simulink model "Part_2_SH_N"  (R2018b)
settings: Solver=VariableStepAuto  StartTime=0.0  StopTime=20.0  MaxStep=0.2  RelTol=1e-3  EnableMultiTasking=on
InitFcn:
  | valve_orifice_area = 0.16;
  | x0 = 0.8;
undefined symbols (not defined in the file): sigbuilder_block
libraries: fl_lib x28, nesl_utility x9, simulink x1
CloseFcn:
  | try,close(h1_sh_power_steering),end
  | clear h1_sh_power_steering
  | try,close(h2_sh_power_steering),end
  | clear h2_sh_power_steering
  | 
  | 
  | clear simlog_sh_power_steering
Description:
  | Power-Assisted Steering Mechanism
  | 
  | Copyright 2008-2018 The MathWorks, Inc.
settings Model: ExtModeAutoUpdateStatusClock=off  Creator=MathWorks  LastModifiedBy=rabia.sehab
settings DataIOCC: LimitDataPoints=on  MaxDataPoints=10000  SaveFormat=Array  SignalLoggingSaveFormat=ModelDataLogs  SignalLoggingName=logsout_sh_power_steering
settings OptimizationCC: ExpressionDepthLimit=2147483647  InitFltsAndDblsToZero=on  LifeSpan=inf
settings DebuggingCC: SaveWithParameterizedLinksMsg=none  UnderspecifiedInitializationDetection=Classic  MergeDetectMultiDrivingBlocksExec=none  SignalResolutionControl=TryResolveAllWithWarning  FcnCallInpInsideContextMsg=warning  AllowSymbolicDim=off  StateNameClashWarn=warning  SFUnexpectedBacktrackingDiag=warning  SFNoUnconditionalDefaultTransitionDiag=warning  SFExecutionAtInitializationDiag=none
settings HardwareCC: ProdBitPerPointer=32  ProdBitPerSizeT=32  ProdBitPerPtrDiffT=32  ProdLargestAtomicFloat=None  ProdIntDivRoundTo=Undefined  ProdEndianess=Unspecified  ProdWordSize=32  ProdHWDeviceType=32-bit Generic
settings ModelReferenceCC: PropagateSignalLabelsOutOfModel=off
settings SFSimCC: SimUseLocalCustomCode=off
settings RTWCC: RTWUseLocalCustomCode=off
settings CodeAppCC: StateflowObjectComments=on
settings GRTTargetCC: TargetFcnLib=ansi_tfl_tmw.mat  TargetLangStandard=C89/C90 (ANSI)  GeneratePreprocessorConditionals=Disable all  CombineOutputUpdateFcns=off  GRTInterface=on
settings ConfigComp: CovMetricSettings=dw  CovHtmlReporting=on  CovSaveCumulativeToWorkspaceVar=on  CovSaveSingleToWorkspaceVar=on  CovExternalEMLEnable=off
settings SimscapeCC: SimscapeLogType=all  SimscapeLogSimulationStatistics=on  SimscapeLogOpenViewer=on  SimscapeLogName=simlog_sh_power_steering  SimscapeLogLimitData=off  SimscapeLogDataHistory=10000

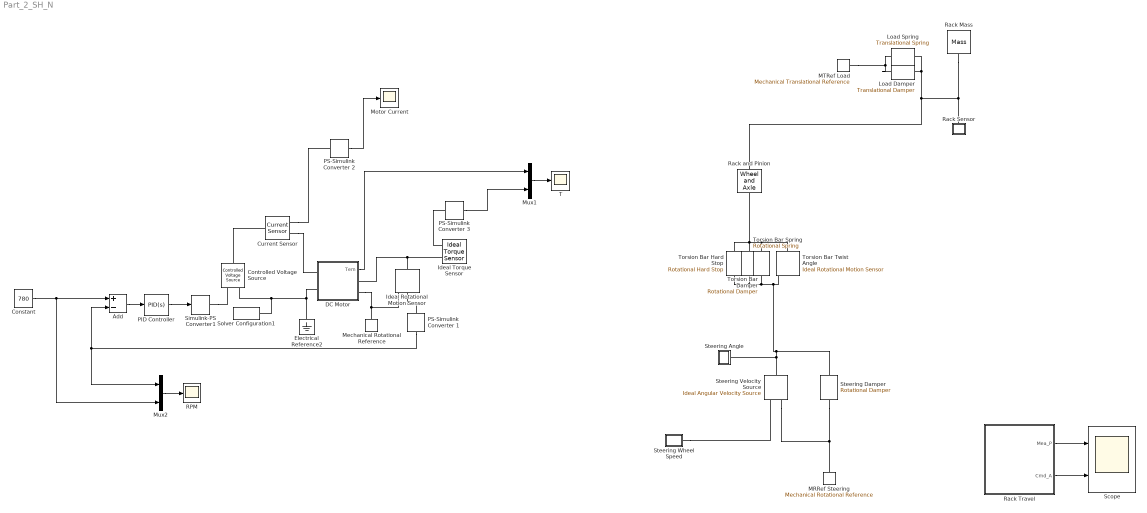
== system Part_2_SH_N ==
  Add : Sum  Inputs=+-
  Constant : Constant  Value=780
  Controlled Voltage Source : fl_lib/Electrical/Electrical Sources/Controlled Voltage Source
  Current Sensor : fl_lib/Electrical/Electrical Sensors/Current Sensor
  DC Motor : Subsystem
  Electrical Reference2 : fl_lib/Electrical/Electrical Elements/Electrical Reference
  Ideal Rotational Motion Sensor : fl_lib/Mechanical/Mechanical Sensors/Ideal Rotational Motion Sensor  offset=0 rad
  Ideal Torque Sensor : fl_lib/Mechanical/Mechanical Sensors/Ideal Torque Sensor
  Load Damper : fl_lib/Mechanical/Translational Elements/Translational Damper  Tag=Factory Generic  D=284 N/(m/s)  v_specify=off  v_priority=High  v=0 m/s  v_nominal_specify=off  v_nominal_unit=m/s  v_nominal_value=1  f_specify=off  f_priority=High  f=0 N  f_nominal_specify=off  f_nominal_unit=N  f_nominal_value=1
  Load Spring : fl_lib/Mechanical/Translational Elements/Translational Spring  Tag=Factory Generic  spr_rate=4450 N/m  v_specify=off  v_priority=High  v=0 m/s  v_nominal_specify=off  v_nominal_unit=m/s  v_nominal_value=1  f_specify=off  f_priority=High  f=0 N  f_nominal_specify=off  f_nominal_unit=N  f_nominal_value=1  x_specify=on  x_priority=High  x=0 m  x_nominal_specify=off  x_nominal_unit=m  x_nominal_value=1
  MRRef Steering : fl_lib/Mechanical/Rotational Elements/Mechanical Rotational Reference  Tag=Factory Generic
  MTRef Load : fl_lib/Mechanical/Translational Elements/Mechanical Translational Reference  Tag=Factory Generic
  Mechanical Rotational Reference : fl_lib/Mechanical/Rotational Elements/Mechanical Rotational Reference
  Motor Current : Scope
  Mux1 : Mux  Inputs=2
  Mux2 : Mux  Inputs=2
  PID Controller : simulink/Continuous/PID Controller  Controller=PID  Form=Parallel  TimeDomain=Continuous-time  SampleTime=-1  IntegratorMethod=Forward Euler  FilterMethod=Forward Euler  ControllerParametersSource=internal  P=0.1  I=10  D=0  UseFilter=on  N=100  TunerSelectOption=Transfer Function Based (PID Tuner App)  InitialConditionSource=internal  InitialConditionForIntegrator=0  InitialConditionForFilter=0  DifferentiatorICPrevScaledInput=0  ExternalReset=none  TrackingMode=off  Kt=1  LimitOutput=off  UpperSaturationLimit=inf  LowerSaturationLimit=-inf  LinearizeAsGain=off  AntiWindupMode=none  Kb=1  POutMin=[]  POutMax=[]  IOutMin=[]  IOutMax=[]  DOutMin=[]  DOutMax=[]  NOutMin=[]  NOutMax=[]  SumOutMin=[]  SumOutMax=[]  SaturationOutMin=[]  SaturationOutMax=[]  PParamMin=[]  PParamMax=[]  IParamMin=[]  IParamMax=[]  DParamMin=[]  DParamMax=[]  NParamMin=[]  NParamMax=[]  KbParamMin=[]  KbParamMax=[]  KtParamMin=[]  KtParamMax=[]  KbOutMin=[]  KbOutMax=[]  KtOutMin=[]  KtOutMax=[]  IntegratorOutMin=[]  IntegratorOutMax=[]  FilterOutMin=[]  FilterOutMax=[]  SumI1OutMin=[]  SumI1OutMax=[]  SumI2OutMin=[]  SumI2OutMax=[]  SumI3OutMin=[]  SumI3OutMax=[]  SumI4OutMin=[]  SumI4OutMax=[]  SumDOutMin=[]  SumDOutMax=[]  DifferentiatorOutMin=[]  DifferentiatorOutMax=[]  FilterDiffOutCoefMin=[]  FilterDiffOutCoefMax=[]  ReciprocalOutMin=[]  ReciprocalOutMax=[]  SumDenOutMin=[]  SumDenOutMax=[]  SumNumOutMin=[]  SumNumOutMax=[]  DivideOutMin=[]  DivideOutMax=[]  IntegratorContinuousStateAttributes=''  IntegratorStateMustResolveToSignalObject=off  IntegratorRTWStateStorageClass=Auto  FilterContinuousStateAttributes=''  FilterStateMustResolveToSignalObject=off  FilterRTWStateStorageClass=Auto  ParallelPVariant=InternalParameters  IdealPVariant=Disabled  IVariant=InternalParameters  DVariant=InternalParameters  IntegratorVariant=Continuous  SatVariant=Disabled  AWVariant=Passthrough  PCopyVariant=Disabled  TRVariant=Disabled  FdbkBlocksVariant=Forward  IdealPFdbkVariant=Disabled  SatFdbkVariant=Disabled  DerivativeFilterVariant=ContFilter  NVariant=InternalParameters  NCopyVariant=Disabled  FilterICVariant=InternalICsFilter  IntegratorICVariant=InternalICs  ExternalResetVariant=Disabled  TRSumVariant=Passthrough  SumFdbkVariant=Disabled  SumVariant=Sum_PID
  PS-Simulink Converter 1 : nesl_utility/PS-Simulink Converter  PhysicalDomain=network_engine_domain  SubClassName=ps_output  LeftPortType=input  RightPortType=output  PseudoPeriodic=off  Frequencies=[]  Unit=rpm  AffineConversion=off
  PS-Simulink Converter 2 : nesl_utility/PS-Simulink Converter  PhysicalDomain=network_engine_domain  SubClassName=ps_output  LeftPortType=input  RightPortType=output  PseudoPeriodic=off  Frequencies=[]  Unit=A  AffineConversion=off
  PS-Simulink Converter 3 : nesl_utility/PS-Simulink Converter  PhysicalDomain=network_engine_domain  SubClassName=ps_output  LeftPortType=input  RightPortType=output  PseudoPeriodic=off  Frequencies=[]  Unit=N*m  AffineConversion=off
  RPM : Scope
  Rack Mass : fl_lib/Mechanical/Translational Elements/Mass  Tag=Factory Generic  mass=114 kg  v_specify=on  v_priority=High  v=0 m/s  v_nominal_specify=off  v_nominal_unit=m/s  v_nominal_value=1  f_specify=off  f_priority=High  f=0 N  f_nominal_specify=off  f_nominal_unit=N  f_nominal_value=1
  Rack Sensor : Subsystem
      mask Display: disp('P');
  Rack Travel : Subsystem
  Rack and Pinion : fl_lib/Mechanical/Mechanisms/Wheel and Axle  Tag=Factory Generic  R=3.8 cm  or=1  t_specify=off  t_priority=High  t=0 N*m  t_nominal_specify=off  t_nominal_unit=N*m  t_nominal_value=1  f_specify=off  f_priority=High  f=0 N  f_nominal_specify=off  f_nominal_unit=N  f_nominal_value=1
      settings: SourceProductName=Simscape
  Scope : Scope  NumInputPorts=2
  Simulink-PS Converter1 : nesl_utility/Simulink-PS Converter  PhysicalDomain=network_engine_domain  SubClassName=ps_input  LeftPortType=input  RightPortType=output  PseudoPeriodic=off  Frequencies=[]  NoiseDistribution=none  NoiseParameters=[]  Unit=1  AffineConversion=off  FilteringAndDerivatives=zero  SimscapeFilterOrder=1  InputFilterTimeConstant=.001  UdotUserProvided=0
  Solver Configuration1 : nesl_utility/Solver Configuration  PhysicalDomain=network_engine_domain  SubClassName=solver  LeftPortType=input  RightPortType=generic  Tones=[]  Harmonics=[]  SimulateNoise=off  Profile=off  UseLocalSampling=off  EnableSwitchedLinearOptims=on  FrequencyDomain=off  UseCCode=off  RelTol=0.001  AbsTol=1e-06  MinStep=1e-09  ToWorkspace=off  RevertToSquareIcSolve=off  NumHomotopyIterations=100  PhasorMode=off  PhasorModeNumHarmonics=1  DoDC=off  ResidualTolerance=1e-9  UseLocalSolver=off  LocalSolverChoice=NE_BACKWARD_EULER_ADVANCER  LocalSolverSampleTime=.001  DoFixedCost=off  MaxNonlinIter=3  MaxModeIter=2  LinearAlgebra=Sparse  EquationFormulation=NE_TIME_EF  DelaysMemoryBudget=1024  AutomaticFiltering=on  FilteringTimeConstant=0.001  PartitionStorageMethod=AS_NEEDED  PartitionMemoryBudget=1024  PartitionMethod=FAST
  Steering Angle : Subsystem
      mask Display: disp('A');
  Steering Damper : fl_lib/Mechanical/Rotational Elements/Rotational Damper  Tag=Factory Generic  D=0.001 N*m/(rad/s)  w_specify=off  w_priority=High  w=0 rad/s  w_nominal_specify=off  w_nominal_unit=rad/s  w_nominal_value=1  t_specify=off  t_priority=High  t=0 N*m  t_nominal_specify=off  t_nominal_unit=N*m  t_nominal_value=1
  Steering Velocity Source : fl_lib/Mechanical/Mechanical Sources/Ideal Angular Velocity Source  Tag=Factory Generic
  Steering Wheel Speed : Subsystem
  T : Scope
  Torsion Bar Hard Stop : fl_lib/Mechanical/Rotational Elements/Rotational Hard Stop  Tag=Factory Generic  upper_bnd=9 deg  lower_bnd=-9 deg  stiff_up=1e+06 N*m/rad  stiff_low=1e6 N*m/rad  D_up=0.01 N*m/(rad/s)  D_low=0.01 N*m/(rad/s)  model=3  transition=0.001 rad  w_specify=off  w_priority=High  w=0 rad/s  w_nominal_specify=off  w_nominal_unit=rad/s  w_nominal_value=1  t_specify=off  t_priority=High  t=0 N*m  t_nominal_specify=off  t_nominal_unit=N*m  t_nominal_value=1  phi_specify=on  phi_priority=High  phi=0 rad  phi_nominal_specify=off  phi_nominal_unit=rad  phi_nominal_value=1
      settings: SourceProductName=Simscape  SourceProductBaseCode=SS
  Torsion Bar Twist Angle : fl_lib/Mechanical/Mechanical Sensors/Ideal Rotational Motion Sensor  Tag=Factory Generic  offset=0 rad
  Torsion Bar Damper : fl_lib/Mechanical/Rotational Elements/Rotational Damper  Tag=Factory Generic  D=0.01 N*m/(rad/s)  w_specify=off  w_priority=High  w=0 rad/s  w_nominal_specify=off  w_nominal_unit=rad/s  w_nominal_value=1  t_specify=off  t_priority=High  t=0 N*m  t_nominal_specify=off  t_nominal_unit=N*m  t_nominal_value=1
  Torsion Bar Spring : fl_lib/Mechanical/Rotational Elements/Rotational Spring  Tag=Factory Generic  spr_rate=10 N*m/rad  w_specify=off  w_priority=High  w=0 rad/s  w_nominal_specify=off  w_nominal_unit=rad/s  w_nominal_value=1  t_specify=off  t_priority=High  t=0 N*m  t_nominal_specify=off  t_nominal_unit=N*m  t_nominal_value=1  phi_specify=on  phi_priority=High  phi=0 rad  phi_nominal_specify=off  phi_nominal_unit=rad  phi_nominal_value=1
      settings: SourceProductName=Simscape
  wires:
  Rack Travel/1(Mea_P) -> Scope/1
  Rack Travel/2(Cmd_A) -> Scope/2
  Add/1 -> PID Controller/1
  PID Controller/1 -> Simulink-PS Converter1/1
  PS-Simulink Converter 1/1 -> Add/2, Mux2/1
  DC Motor/1(Tem) -> Mux1/1
  PS-Simulink Converter 3/1 -> Mux1/2
  Mux2/1 -> RPM/1
  Mux1/1 -> T/1
  Constant/1 -> Mux2/2, Add/1
  PS-Simulink Converter 2/1 -> Motor Current/1
  connections:
  Steering Velocity Source/RConn2 -- Steering Damper/RConn1 -- MRRef Steering/LConn1
  Steering Velocity Source/LConn1 -- Steering Damper/LConn1 -- Torsion Bar Spring/RConn1 -- Torsion Bar Hard Stop/RConn1 -- Torsion Bar Damper/RConn1 -- Torsion Bar Twist Angle/RConn1 -- Steering Angle/LConn1
  Rack and Pinion/LConn1 -- Torsion Bar Twist Angle/LConn1 -- Torsion Bar Spring/LConn1 -- Torsion Bar Hard Stop/LConn1 -- Torsion Bar Damper/LConn1
  Rack Mass/LConn1 -- Load Spring/LConn1 -- Load Damper/LConn1 -- Rack and Pinion/RConn1 -- Rack Sensor/LConn1
  MTRef Load/LConn1 -- Load Spring/RConn1 -- Load Damper/RConn1
  Steering Wheel Speed/RConn1 -- Steering Velocity Source/RConn1
  Ideal Torque Sensor/RConn1 -- Ideal Rotational Motion Sensor/LConn1 -- DC Motor/RConn1
  Solver Configuration1/RConn1 -- Electrical Reference2/LConn1 -- DC Motor/LConn2 -- Controlled Voltage Source/RConn2
  Ideal Rotational Motion Sensor/RConn1 -- DC Motor/RConn2 -- Mechanical Rotational Reference/LConn1
  Current Sensor/RConn2 -- DC Motor/LConn1
  Ideal Rotational Motion Sensor/RConn2 -- PS-Simulink Converter 1/LConn1
  Simulink-PS Converter1/RConn1 -- Controlled Voltage Source/RConn1
  Controlled Voltage Source/LConn1 -- Current Sensor/LConn1
  Ideal Torque Sensor/RConn2 -- PS-Simulink Converter 3/LConn1
  Current Sensor/RConn1 -- PS-Simulink Converter 2/LConn1

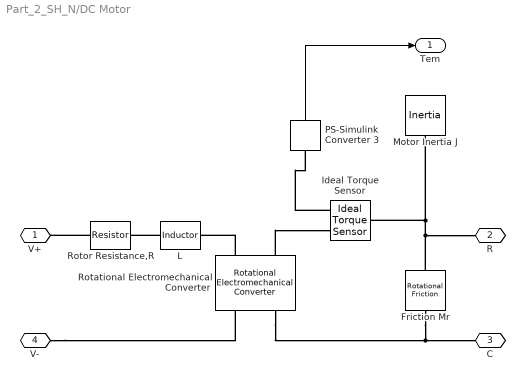
== system Part_2_SH_N/DC Motor ==
  Friction Mr : fl_lib/Mechanical/Rotational Elements/Rotational Friction  brkwy_trq=.5 N*m  brkwy_vel=0.03347 rad/s  Col_trq=.5 N*m  visc_coef=1e-4 N*m/rpm  w_specify=off  w_priority=None  w=0 rad/s  w_nominal_specify=off  w_nominal_unit=rad/s  w_nominal_value=1  t_specify=off  t_priority=None  t=0 N*m  t_nominal_specify=off  t_nominal_unit=N*m  t_nominal_value=1
      settings: SourceProductName=Simscape
  Ideal Torque Sensor : fl_lib/Mechanical/Mechanical Sensors/Ideal Torque Sensor
  L : fl_lib/Electrical/Electrical Elements/Inductor  l=.01 H  r=0 Ohm  g=1e-09 1/Ohm  i_specify=off  i_priority=None  i=0 A  i_nominal_specify=off  i_nominal_unit=A  i_nominal_value=1  v_specify=off  v_priority=None  v=0 V  v_nominal_specify=off  v_nominal_unit=V  v_nominal_value=1  i_L_specify=on  i_L_priority=High  i_L=0 A  i_L_nominal_specify=off  i_L_nominal_unit=A  i_L_nominal_value=1
  Motor Inertia J : fl_lib/Mechanical/Rotational Elements/Inertia  inertia=1e-4 kg*m^2  w_specify=on  w_priority=High  w=0 rad/s  w_nominal_specify=off  w_nominal_unit=rad/s  w_nominal_value=1  t_specify=off  t_priority=None  t=0 N*m  t_nominal_specify=off  t_nominal_unit=N*m  t_nominal_value=1
  PS-Simulink Converter 3 : nesl_utility/PS-Simulink Converter  PhysicalDomain=network_engine_domain  SubClassName=ps_output  LeftPortType=input  RightPortType=output  PseudoPeriodic=off  Frequencies=[]  Unit=N*m  AffineConversion=off
  Rotational Electromechanical Converter : fl_lib/Electrical/Electrical Elements/Rotational Electromechanical Converter  K=.5 V/(rad/s)  i_specify=off  i_priority=None  i=0 A  i_nominal_specify=off  i_nominal_unit=A  i_nominal_value=1  v_specify=off  v_priority=None  v=0 V  v_nominal_specify=off  v_nominal_unit=V  v_nominal_value=1  t_specify=off  t_priority=None  t=0 N*m  t_nominal_specify=off  t_nominal_unit=N*m  t_nominal_value=1  w_specify=off  w_priority=None  w=0 rad/s  w_nominal_specify=off  w_nominal_unit=rad/s  w_nominal_value=1
      settings: SourceProductName=Simscape
  Rotor Resistance,R : fl_lib/Electrical/Electrical Elements/Resistor  Tag=Factory Generic  R=1.15 Ohm  i_specify=off  i_priority=None  i=0 A  i_nominal_specify=off  i_nominal_unit=A  i_nominal_value=1  v_specify=off  v_priority=None  v=0 V  v_nominal_specify=off  v_nominal_unit=V  v_nominal_value=1
  V+ : PMIOPort  Side=Left
  R : PMIOPort  Port=2  Side=Right
  C : PMIOPort  Port=3  Side=Right
  V- : PMIOPort  Port=4  Side=Left
  Tem : Outport  VectorParamsAs1DForOutWhenUnconnected=off
  wires:
  PS-Simulink Converter 3/1 -> Tem/1
  connections:
  Rotational Electromechanical Converter/LConn1 -- L/RConn1
  V-/RConn1 -- Rotational Electromechanical Converter/RConn1
  Rotor Resistance,R/LConn1 -- V+/RConn1
  L/LConn1 -- Rotor Resistance,R/RConn1
  Friction Mr/LConn1 -- R/RConn1 -- Motor Inertia J/LConn1 -- Ideal Torque Sensor/LConn1
  Rotational Electromechanical Converter/RConn2 -- C/RConn1 -- Friction Mr/RConn1
  Rotational Electromechanical Converter/LConn2 -- Ideal Torque Sensor/RConn1
  Ideal Torque Sensor/RConn2 -- PS-Simulink Converter 3/LConn1

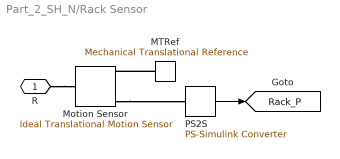
== system Part_2_SH_N/Rack Sensor ==
  MTRef : fl_lib/Mechanical/Translational Elements/Mechanical Translational Reference  Tag=Factory Generic
  Motion Sensor : fl_lib/Mechanical/Mechanical Sensors/Ideal Translational Motion Sensor  Tag=Factory Generic  offset=0 m
  PS2S : nesl_utility/PS-Simulink Converter  PhysicalDomain=network_engine_domain  SubClassName=ps_output  LeftPortType=input  RightPortType=output  PseudoPeriodic=off  Frequencies=[]  Unit=1  AffineConversion=off
  R : PMIOPort  Side=Left
  tag scope: Rack_P=global
  wires:
  PS2S/1 -> [Rack_P]
  connections:
  R/RConn1 -- Motion Sensor/LConn1
  Motion Sensor/RConn3 -- PS2S/LConn1
  MTRef/LConn1 -- Motion Sensor/RConn1

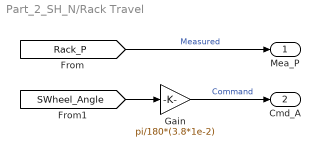
== system Part_2_SH_N/Rack Travel ==
  Gain : Gain  Gain=pi/180*(3.8*1e-2)
  Mea_P : Outport  VectorParamsAs1DForOutWhenUnconnected=off
  Cmd_A : Outport  Port=2  VectorParamsAs1DForOutWhenUnconnected=off
  wires:
  [Rack_P] -> Mea_P/1  "Measured"
  [SWheel_Angle] -> Gain/1
  Gain/1 -> Cmd_A/1  "Command"

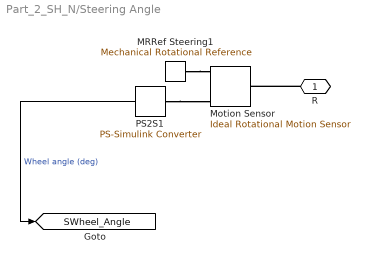
== system Part_2_SH_N/Steering Angle ==
  MRRef Steering1 : fl_lib/Mechanical/Rotational Elements/Mechanical Rotational Reference  Tag=Factory Generic
  Motion Sensor : fl_lib/Mechanical/Mechanical Sensors/Ideal Rotational Motion Sensor  Tag=Factory Generic  offset=0 rad
  PS2S1 : nesl_utility/PS-Simulink Converter  PhysicalDomain=network_engine_domain  SubClassName=ps_output  LeftPortType=input  RightPortType=output  PseudoPeriodic=off  Frequencies=[]  Unit=deg  AffineConversion=off
  R : PMIOPort  Side=Left
  tag scope: SWheel_Angle=global
  wires:
  PS2S1/1 -> [SWheel_Angle]  "Wheel angle (deg)"
  connections:
  PS2S1/LConn1 -- Motion Sensor/RConn3
  R/RConn1 -- Motion Sensor/LConn1
  MRRef Steering1/LConn1 -- Motion Sensor/RConn1

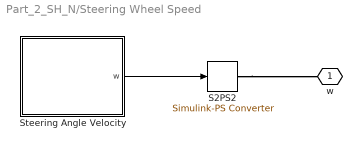
== system Part_2_SH_N/Steering Wheel Speed ==
  S2PS2 : nesl_utility/Simulink-PS Converter  PhysicalDomain=network_engine_domain  SubClassName=ps_input  LeftPortType=input  RightPortType=output  PseudoPeriodic=off  Frequencies=[]  NoiseDistribution=none  NoiseParameters=[]  Unit=rpm  AffineConversion=off  FilteringAndDerivatives=zero  SimscapeFilterOrder=1  InputFilterTimeConstant=.001  UdotUserProvided=0
  Steering Angle Velocity : Subsystem  Tag=STV Subsys  LoadFcn=sigbuilder_block('load');  StartFcn=sigbuilder_block('start');  StopFcn=sigbuilder_block('stop');  ClipboardFcn=sigbuilder_block('clipboard');  mask(Sigbuilder block){tuvar=[0:10]}
      mask help: Sigbuilder GUI
      mask init:
      | if ~strcmp(get_param(bdroot(gcbh),'SimulationStatus'),'stopped') tuvar = sigbuilder_block('maskInit'); end
      settings: CopyFcn=sigbuilder_block('copy');  DeleteFcn=sigbuilder_block('delete');  ModelCloseFcn=sigbuilder_block('modelClose');  PreSaveFcn=sigbuilder_block('preSave');  PauseFcn=sigbuilder_block('pause')  ContinueFcn=sigbuilder_block('continue')  NameChangeFcn=sigbuilder_block('namechange');  OpenFcn=sigbuilder_block('open',[437.6 199.2 550.4 400 ]);  CloseFcn=sigbuilder_block('close');
      mask Display: plot(0, 0, 100, 100,[2, 2, 32, 32, 2], [68, 8, 8, 68, 68],[32, 2], [38, 38], [32, 19, 2],[53, 60, 44], [32, 17, 17, 2],[16, 16, 31, 31]);txt = getActiveGroup(gcbh);text(2, 100, txt,'verticalAlignment', 'top');
  w : PMIOPort  Side=Right
  wires:
  Steering Angle Velocity/1(w) -> S2PS2/1
  connections:
  S2PS2/RConn1 -- w/RConn1

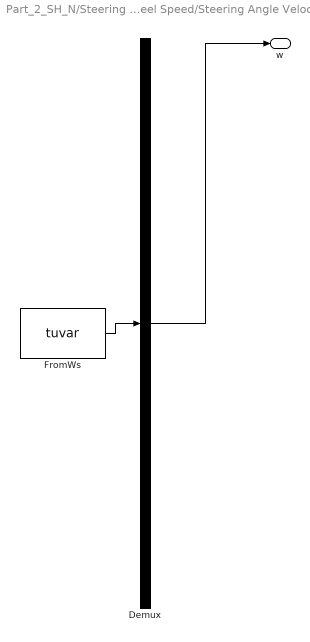
== system Part_2_SH_N/Steering Wheel Speed/Steering Angle Velocity ==
  Demux : Demux  Tag=STV Demux  Outputs=1
  FromWs : FromWorkspace  Tag=STV FromWs  VariableName=tuvar  SampleTime=0
      SigBuilderData=|
      | common.afterFinalStr = 'Extrapolate'
      | common.sampleTime = 0
      | dataSet.timeRange = [0 20]
      | dataSet.name = 'Group 1'
      | sbobj.Groups.Name = 'Group 1'
      | sbobj.Groups.Signals.Name = 'w'
      | sbobj.Groups.Signals.XData = [0 1.96 2.4 4.05 4.5 5.95 6.75 8.05 8.4 10 10.35 11.7 12 13.85 14.2 15.7 15.95 20]
      | sbobj.Groups.Signals.YData = [0 0 0.99 1 0 0 -1 -1 0 0 -1 -0.99 0 0 1 1 0 0]
      | sbobj.Groups.TimeRange = [0 20]
  w : Outport  Tag=STV Outport  VectorParamsAs1DForOutWhenUnconnected=off
  wires:
  FromWs/1 -> Demux/1
  Demux/1 -> w/1
